simulink model "straight_TMS4_PH_ORC_OL"  (R2022a)
settings: Solver=VariableStepAuto  StartTime=0.0  StopTime=3000  RelTol=1e-3
model workspace: external: MATLAB File parameters_straight.m (data not in the file)
undefined symbols (not defined in the file): BoP, cf, clch, clnt, const, h2o, htr, HX_ORCph, HX_ph, ORCph, pemel, prch
libraries: fl_lib x67, nesl_utility x23, SimscapeFluids_lib x7, slpidlib x4
(part 3 of 3)

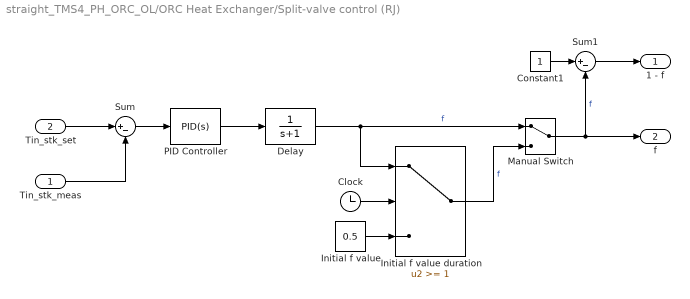
== system straight_TMS4_PH_ORC_OL/ORC Heat Exchanger/Split-valve control (RJ) ==
  Tin_stk_meas : Inport
  Tin_stk_set : Inport  Port=2
  Clock : Clock
  Constant1 : Constant
  Delay : TransferFcn  Denominator=[1 1]
  Initial f value : Constant  Value=0.5
  Initial f value duration : Switch  Threshold=1  SaturateOnIntegerOverflow=off  InputSameDT=off
  Manual Switch : ManualSwitch
  PID Controller : slpidlib/PID Controller  Controller=PID  Form=Ideal  TimeDomain=Continuous-time  UseExternalTs=off  SampleTime=-1  IntegratorMethod=Forward Euler  FilterMethod=Forward Euler  ControllerParametersSource=internal  P=-0.555708182490552  I=0.95717123634426  UseKiTs=off  D=0.096496205335411  N=3.15255555770467  UseFilter=on  TunerSelectOption=Transfer Function Based (PID Tuner App)  InitialConditionSource=internal  InitialConditionForIntegrator=0  InitialConditionForFilter=0  DifferentiatorICPrevScaledInput=0  ExternalReset=none  TrackingMode=off  Kt=1  LimitOutput=on  SatLimitsSource=internal  UpperSaturationLimit=1  LowerSaturationLimit=0  LinearizeAsGain=on  AntiWindupMode=back-calculation  Kb=0.1  POutMin=[]  POutMax=[]  IOutMin=[]  IOutMax=[]  DOutMin=[]  DOutMax=[]  NOutMin=[]  NOutMax=[]  SumOutMin=[]  SumOutMax=[]  SaturationOutMin=[]  SaturationOutMax=[]  PParamMin=[]  PParamMax=[]  IParamMin=[]  IParamMax=[]  DParamMin=[]  DParamMax=[]  NParamMin=[]  NParamMax=[]  KbParamMin=[]  KbParamMax=[]  KtParamMin=[]  KtParamMax=[]  KbOutMin=[]  KbOutMax=[]  KtOutMin=[]  KtOutMax=[]  IntegratorOutMin=[]  IntegratorOutMax=[]  FilterOutMin=[]  FilterOutMax=[]  SumI1OutMin=[]  SumI1OutMax=[]  SumI2OutMin=[]  SumI2OutMax=[]  SumI3OutMin=[]  SumI3OutMax=[]  SumI4OutMin=[]  SumI4OutMax=[]  SumDOutMin=[]  SumDOutMax=[]  DifferentiatorOutMin=[]  DifferentiatorOutMax=[]  FilterDiffOutCoefMin=[]  FilterDiffOutCoefMax=[]  ReciprocalOutMin=[]  ReciprocalOutMax=[]  SumDenOutMin=[]  SumDenOutMax=[]  SumNumOutMin=[]  SumNumOutMax=[]  DivideOutMin=[]  DivideOutMax=[]  UdiffTsProdOutMin=[]  UdiffTsProdOutMax=[]  NTsProdOutMin=[]  NTsProdOutMax=[]  UintegralTsProdOutMin=[]  UintegralTsProdOutMax=[]  UngainTsProdOutMin=[]  UngainTsProdOutMax=[]  IntegratorContinuousStateAttributes=''  IntegratorStateMustResolveToSignalObject=off  IntegratorRTWStateStorageClass=Auto  FilterContinuousStateAttributes=''  FilterStateMustResolveToSignalObject=off  FilterRTWStateStorageClass=Auto  ParallelPVariant=Passthrough  IdealPVariant=InternalParameters  IVariant=InternalParameters  DVariant=InternalParameters  IntegratorVariant=Continuous  SatVariant=Enabled  AWVariant=BackCalculation  PCopyVariant=Disabled  TRVariant=Disabled  FdbkBlocksVariant=Forward  IdealPFdbkVariant=Disabled  SatFdbkVariant=Disabled  DerivativeFilterVariant=ContFilter  NVariant=InternalParameters  NCopyVariant=Disabled  FilterICVariant=InternalICsFilter  IntegratorICVariant=InternalICs  ExternalResetVariant=Disabled  TRSumVariant=Passthrough  SumFdbkVariant=Disabled  SumVariant=Sum_PID  TsampFilterVariant=InternalTs  TsampNgainVariant=Passthrough  TsampIntegralVariant=Passthrough  ExternalSaturationOutDataTypeStr=Inherit: Same as second input  aMode=0
  Sum : Sum  Inputs=|+-
  Sum1 : Sum  Inputs=|+-
  1 - f : Outport
  f : Outport  Port=2
  wires:
  Sum1/1 -> 1 - f/1
  Sum/1 -> PID Controller/1
  Tin_stk_set/1 -> Sum/1
  Tin_stk_meas/1 -> Sum/2
  PID Controller/1 -> Delay/1
  Constant1/1 -> Sum1/1
  Initial f value/1 -> Initial f value duration/3
  Clock/1 -> Initial f value duration/2
  Delay/1 -> Initial f value duration/1, Manual Switch/1  "f"
  Initial f value duration/1 -> Manual Switch/2  "f"
  Manual Switch/1 -> Sum1/2, f/1  "f"

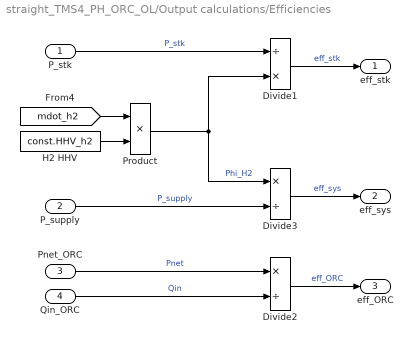
== system straight_TMS4_PH_ORC_OL/Output calculations/Efficiencies ==
  P_stk : Inport
  P_supply : Inport  Port=2
  Pnet_ORC : Inport  Port=3
  Qin_ORC : Inport  Port=4
  Divide1 : Product  Inputs=/*
  Divide2 : Product  Inputs=*/
  Divide3 : Product  Inputs=*/
  H2 HHV : Constant  Value=const.HHV_h2
  Product : Product
  eff_stk : Outport
  eff_sys : Outport  Port=2
  eff_ORC : Outport  Port=3
  wires:
  Pnet_ORC/1 -> Divide2/1  "Pnet"
  Qin_ORC/1 -> Divide2/2  "Qin"
  Divide2/1 -> eff_ORC/1  "eff_ORC"
  [mdot_h2] -> Product/1
  Divide1/1 -> eff_stk/1  "eff_stk"
  Divide3/1 -> eff_sys/1  "eff_sys"
  P_stk/1 -> Divide1/1  "P_stk"
  H2 HHV/1 -> Product/2
  Product/1 -> Divide1/2, Divide3/1  "Phi_H2"
  P_supply/1 -> Divide3/2  "P_supply"

== system straight_TMS4_PH_ORC_OL/Output calculations/Heat transfer ==
  Abs : Abs  SaturateOnIntegerOverflow=off
  Mux1 : Mux  Inputs=3
  Subtract : Sum  Inputs=-+
  Subtract1 : Sum  Inputs=-+
  Subtract2 : Sum  Inputs=-+
  Qin_ORC : Outport
  Qclnt_i : Outport  Port=2
  wires:
  Abs/1 -> Qin_ORC/1  "Qdot_ORC_in"
  Mux1/1 -> Qclnt_i/1  "Qdot_i"
  [Phi_clnt_rjOut] -> Subtract2/2  "Phi_clnt_rjOut"
  Subtract2/1 -> Abs/1, Mux1/3  "Qdot_clnt_rj"
  [Phi_clnt_stkOut] -> Subtract/2, Subtract1/1  "Phi_clnt_stkOut"
  Subtract1/1 -> Mux1/2  "Qdot_clnt_PH"
  Subtract/1 -> Mux1/1  "Qdot_clnt_stk"
  [Phi_clnt_phOut] -> Subtract2/1, Subtract1/2  "Phi_clnt_phOut"
  [Phi_clnt_stkIn] -> Subtract/1  "Phi_clnt_stkIn"

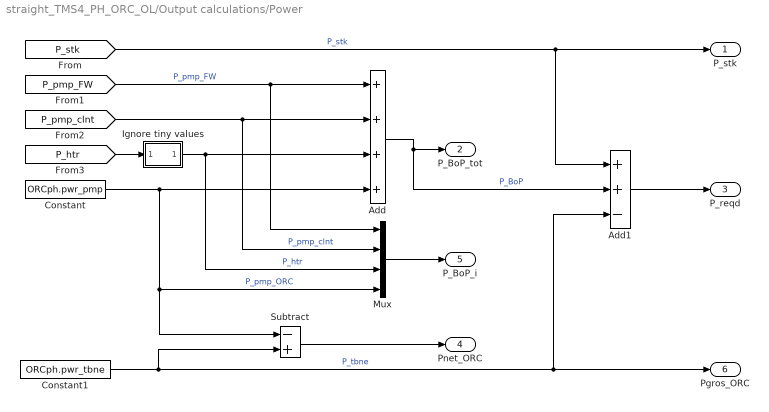
== system straight_TMS4_PH_ORC_OL/Output calculations/Power ==
  Add : Sum  Inputs=++++
  Add1 : Sum  Inputs=++-
  Constant : Constant  Value=ORCph.pwr_pmp
  Constant1 : Constant  Value=ORCph.pwr_tbne
  Ignore tiny values : Subsystem
  Mux : Mux
  Subtract : Sum  Inputs=-+
  P_stk : Outport
  P_BoP_tot : Outport  Port=2
  P_reqd : Outport  Port=3
  Pnet_ORC : Outport  Port=4
  P_BoP_i : Outport  Port=5
  Pgros_ORC : Outport  Port=6
  wires:
  [P_pmp_clnt] -> Mux/2, Add/2  "P_pmp_clnt"
  Add/1 -> Add1/2, P_BoP_tot/1  "P_BoP"
  [P_pmp_FW] -> Mux/1, Add/1  "P_pmp_FW"
  Mux/1 -> P_BoP_i/1
  [P_stk] -> P_stk/1, Add1/1  "P_stk"
  Constant1/1 -> Pgros_ORC/1, Add1/3, Subtract/2  "P_tbne"
  Add1/1 -> P_reqd/1
  Constant/1 -> Mux/4, Subtract/1, Add/4  "P_pmp_ORC"
  Subtract/1 -> Pnet_ORC/1
  Ignore tiny values/1(Out1) -> Mux/3, Add/3  "P_htr"
  [P_htr] -> Ignore tiny values/1(In1)

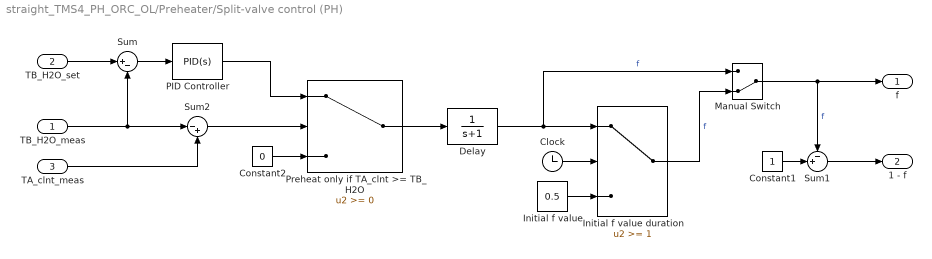
== system straight_TMS4_PH_ORC_OL/Preheater/Split-valve control (PH) ==
  TB_H2O_meas : Inport
  TB_H2O_set : Inport  Port=2
  TA_clnt_meas : Inport  Port=3
  Clock : Clock
  Constant1 : Constant
  Constant2 : Constant  Value=0
  Delay : TransferFcn  Denominator=[1 1]
  Initial f value : Constant  Value=0.5
  Initial f value duration : Switch  Threshold=1  SaturateOnIntegerOverflow=off  InputSameDT=off
  Manual Switch : ManualSwitch  CurrentSetting=0
  PID Controller : slpidlib/PID Controller  Controller=PID  Form=Ideal  TimeDomain=Continuous-time  UseExternalTs=off  SampleTime=-1  IntegratorMethod=Forward Euler  FilterMethod=Forward Euler  ControllerParametersSource=internal  P=25.8351394776647  I=0.0997386043902792  UseKiTs=off  D=1.11064827090151  N=1491.94252746946  UseFilter=on  TunerSelectOption=Transfer Function Based (PID Tuner App)  InitialConditionSource=internal  InitialConditionForIntegrator=0  InitialConditionForFilter=0  DifferentiatorICPrevScaledInput=0  ExternalReset=none  TrackingMode=off  Kt=1  LimitOutput=on  SatLimitsSource=internal  UpperSaturationLimit=1  LowerSaturationLimit=0  LinearizeAsGain=on  AntiWindupMode=back-calculation  Kb=0.1  POutMin=[]  POutMax=[]  IOutMin=[]  IOutMax=[]  DOutMin=[]  DOutMax=[]  NOutMin=[]  NOutMax=[]  SumOutMin=[]  SumOutMax=[]  SaturationOutMin=[]  SaturationOutMax=[]  PParamMin=[]  PParamMax=[]  IParamMin=[]  IParamMax=[]  DParamMin=[]  DParamMax=[]  NParamMin=[]  NParamMax=[]  KbParamMin=[]  KbParamMax=[]  KtParamMin=[]  KtParamMax=[]  KbOutMin=[]  KbOutMax=[]  KtOutMin=[]  KtOutMax=[]  IntegratorOutMin=[]  IntegratorOutMax=[]  FilterOutMin=[]  FilterOutMax=[]  SumI1OutMin=[]  SumI1OutMax=[]  SumI2OutMin=[]  SumI2OutMax=[]  SumI3OutMin=[]  SumI3OutMax=[]  SumI4OutMin=[]  SumI4OutMax=[]  SumDOutMin=[]  SumDOutMax=[]  DifferentiatorOutMin=[]  DifferentiatorOutMax=[]  FilterDiffOutCoefMin=[]  FilterDiffOutCoefMax=[]  ReciprocalOutMin=[]  ReciprocalOutMax=[]  SumDenOutMin=[]  SumDenOutMax=[]  SumNumOutMin=[]  SumNumOutMax=[]  DivideOutMin=[]  DivideOutMax=[]  UdiffTsProdOutMin=[]  UdiffTsProdOutMax=[]  NTsProdOutMin=[]  NTsProdOutMax=[]  UintegralTsProdOutMin=[]  UintegralTsProdOutMax=[]  UngainTsProdOutMin=[]  UngainTsProdOutMax=[]  IntegratorContinuousStateAttributes=''  IntegratorStateMustResolveToSignalObject=off  IntegratorRTWStateStorageClass=Auto  FilterContinuousStateAttributes=''  FilterStateMustResolveToSignalObject=off  FilterRTWStateStorageClass=Auto  ParallelPVariant=Passthrough  IdealPVariant=InternalParameters  IVariant=InternalParameters  DVariant=InternalParameters  IntegratorVariant=Continuous  SatVariant=Enabled  AWVariant=BackCalculation  PCopyVariant=Disabled  TRVariant=Disabled  FdbkBlocksVariant=Forward  IdealPFdbkVariant=Disabled  SatFdbkVariant=Disabled  DerivativeFilterVariant=ContFilter  NVariant=InternalParameters  NCopyVariant=Disabled  FilterICVariant=InternalICsFilter  IntegratorICVariant=InternalICs  ExternalResetVariant=Disabled  TRSumVariant=Passthrough  SumFdbkVariant=Disabled  SumVariant=Sum_PID  TsampFilterVariant=InternalTs  TsampNgainVariant=Passthrough  TsampIntegralVariant=Passthrough  ExternalSaturationOutDataTypeStr=Inherit: Same as second input  aMode=0
  "Preheat only if TA_clnt >= TB_H2O " : Switch  SaturateOnIntegerOverflow=off  InputSameDT=off
  Sum : Sum  Inputs=|+-
  Sum1 : Sum  Inputs=-+|
  Sum2 : Sum  Inputs=|-+
  f : Outport
  1 - f : Outport  Port=2
  wires:
  TB_H2O_meas/1 -> Sum2/1, Sum/2
  TB_H2O_set/1 -> Sum/1
  Sum/1 -> PID Controller/1
  PID Controller/1 -> "Preheat only if TA_clnt >= TB_H2O "/1
  Sum1/1 -> 1 - f/1
  TA_clnt_meas/1 -> Sum2/2
  Sum2/1 -> "Preheat only if TA_clnt >= TB_H2O "/2
  Constant2/1 -> "Preheat only if TA_clnt >= TB_H2O "/3
  Constant1/1 -> Sum1/2
  Clock/1 -> Initial f value duration/2
  Initial f value/1 -> Initial f value duration/3
  "Preheat only if TA_clnt >= TB_H2O "/1 -> Delay/1
  Delay/1 -> Initial f value duration/1, Manual Switch/1  "f"
  Initial f value duration/1 -> Manual Switch/2  "f"
  Manual Switch/1 -> f/1, Sum1/1  "f"

== system straight_TMS4_PH_ORC_OL/Preheater/Temp sensor (H2O_B) ==
  Absolute Reference (TL)1 : fl_lib/Thermal Liquid/Elements/Absolute Reference (TL)
      settings: SourceProductBaseCode=PW,SS,VE
  PS Terminator1 : fl_lib/Physical Signals/Sinks/PS Terminator
      settings: SourceProductBaseCode=PW,SS,VE
  PS-Simulink Converter1 : nesl_utility/PS-Simulink Converter  PhysicalDomain=network_engine_domain  SubClassName=ps_output  LeftPortType=input  RightPortType=output  PseudoPeriodic=off  Frequencies=[]  VectorFormat=1-D array  Unit=K  AffineConversion=off
      settings: SourceProductBaseCode=SS,PW,VE
  Pressure & Temperature Sensor (TL)1 : fl_lib/Thermal Liquid/Sensors/Pressure & Temperature Sensor (TL)
      settings: SourceProductBaseCode=PW,SS,VE  InternalSimscapePortConfiguration="{\"Bottom\":[],\"Left\":[{\"id\":\"A\",\"label\":\"A\",\"type\":\"foundation.thermal_liquid.thermal_liquid\"}],\"Right\":[{\"id\":\"B\",\"label\":\"B\",\"type\":\"foundation.thermal_liquid.thermal_liquid\"},{\"id\":\"P\",\"label\":\"P\",\"type\":\"output\"},{\"id\":\"T\",\"label\":\"T\",\"type\":\"output\"}],\"Top\":[]}"
  A : PMIOPort  Side=Left
  T : Outport
  wires:
  PS-Simulink Converter1/1 -> T/1
  connections:
  Pressure & Temperature Sensor (TL)1/RConn3 -- PS-Simulink Converter1/LConn1
  Pressure & Temperature Sensor (TL)1/RConn2 -- PS Terminator1/LConn1
  Pressure & Temperature Sensor (TL)1/LConn1 -- A/RConn1
  Pressure & Temperature Sensor (TL)1/RConn1 -- Absolute Reference (TL)1/LConn1

== system straight_TMS4_PH_ORC_OL/Preheater/Temp sensor (clnt_A) ==
  Absolute Reference (TL)1 : fl_lib/Thermal Liquid/Elements/Absolute Reference (TL)
      settings: SourceProductBaseCode=PW,SS,VE
  PS Terminator1 : fl_lib/Physical Signals/Sinks/PS Terminator
      settings: SourceProductBaseCode=PW,SS,VE
  PS-Simulink Converter1 : nesl_utility/PS-Simulink Converter  PhysicalDomain=network_engine_domain  SubClassName=ps_output  LeftPortType=input  RightPortType=output  PseudoPeriodic=off  Frequencies=[]  VectorFormat=1-D array  Unit=K  AffineConversion=off
      settings: SourceProductBaseCode=SS,PW,VE
  Pressure & Temperature Sensor (TL)1 : fl_lib/Thermal Liquid/Sensors/Pressure & Temperature Sensor (TL)
      settings: SourceProductBaseCode=PW,SS,VE  InternalSimscapePortConfiguration="{\"Bottom\":[],\"Left\":[{\"id\":\"A\",\"label\":\"A\",\"type\":\"foundation.thermal_liquid.thermal_liquid\"}],\"Right\":[{\"id\":\"B\",\"label\":\"B\",\"type\":\"foundation.thermal_liquid.thermal_liquid\"},{\"id\":\"P\",\"label\":\"P\",\"type\":\"output\"},{\"id\":\"T\",\"label\":\"T\",\"type\":\"output\"}],\"Top\":[]}"
  A : PMIOPort  Side=Left
  T : Outport
  wires:
  PS-Simulink Converter1/1 -> T/1
  connections:
  Pressure & Temperature Sensor (TL)1/RConn1 -- Absolute Reference (TL)1/LConn1
  Pressure & Temperature Sensor (TL)1/LConn1 -- A/RConn1
  Pressure & Temperature Sensor (TL)1/RConn2 -- PS Terminator1/LConn1
  Pressure & Temperature Sensor (TL)1/RConn3 -- PS-Simulink Converter1/LConn1

== system straight_TMS4_PH_ORC_OL/Output calculations/Power/Ignore tiny values ==
  In1 : Inport
  Constant2 : Constant  Value=0
  Switch : Switch  Threshold=0.1  SaturateOnIntegerOverflow=off  InputSameDT=off
  Out1 : Outport
  wires:
  In1/1 -> Switch/2, Switch/1
  Constant2/1 -> Switch/3
  Switch/1 -> Out1/1  "P_htr"
